simulink library "nonlinearPlant_ul"  (R2018a)
settings: Solver=VariableStepAuto  StartTime=0.0  StopTime=10.0  RelTol=1e-3
values from neighbouring files (symbols this model uses):
  headingTimeConstant_s = 1    [nonlinearPlant_init.m]
  initialHeading_deg = 0    [nonlinearPlant_init.m]
  initialSpeed_mPs = 0    [nonlinearPlant_init.m]
  speedTimeConstant_s = 1    [nonlinearPlant_init.m]
settings Model: Creator=mcobb  LastModifiedBy=mcobb

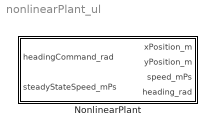
== system nonlinearPlant_ul ==
  NonlinearPlant : Subsystem

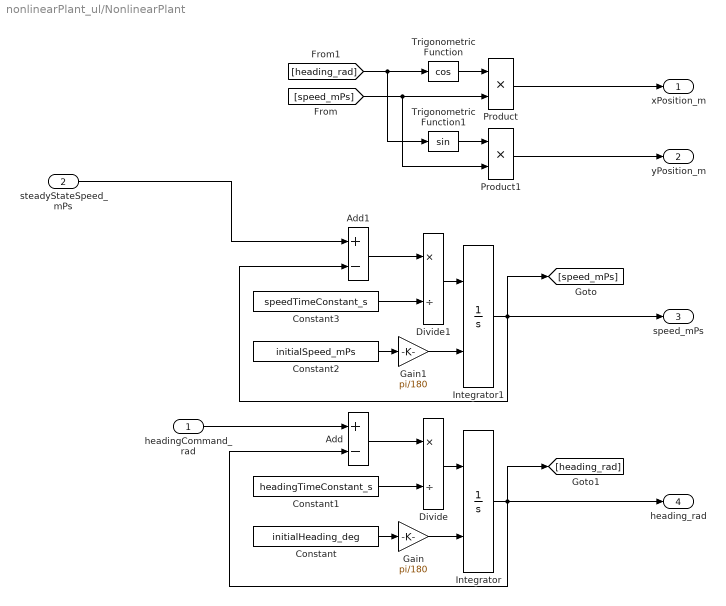
== system nonlinearPlant_ul/NonlinearPlant ==
  headingCommand_rad : Inport
  steadyStateSpeed_mPs : Inport  Port=2
  Add : Sum  Inputs=+-
  Add1 : Sum  Inputs=+-
  Constant : Constant  Value=initialHeading_deg
  Constant1 : Constant  Value=headingTimeConstant_s
  Constant2 : Constant  Value=initialSpeed_mPs
  Constant3 : Constant  Value=speedTimeConstant_s
  Divide : Product  Inputs=*/
  Divide1 : Product  Inputs=*/
  Gain : Gain  Gain=pi/180
  Gain1 : Gain  Gain=pi/180
  Integrator : Integrator  InitialConditionSource=external
  Integrator1 : Integrator  InitialConditionSource=external
  Product : Product
  Product1 : Product
  Trigonometric Function : Trigonometry  Operator=cos
  Trigonometric Function1 : Trigonometry
  xPosition_m : Outport
  yPosition_m : Outport  Port=2
  speed_mPs : Outport  Port=3
  heading_rad : Outport  Port=4
  wires:
  Trigonometric Function/1 -> Product/1
  [heading_rad] -> Trigonometric Function/1, Trigonometric Function1/1
  Product/1 -> xPosition_m/1
  Product1/1 -> yPosition_m/1
  [speed_mPs] -> Product1/2, Product/2
  Trigonometric Function1/1 -> Product1/1
  Constant/1 -> Gain/1
  Gain/1 -> Integrator/2
  Constant1/1 -> Divide/2
  Add/1 -> Divide/1
  Divide/1 -> Integrator/1
  Integrator/1 -> [heading_rad], heading_rad/1, Add/2
  headingCommand_rad/1 -> Add/1
  steadyStateSpeed_mPs/1 -> Add1/1
  Integrator1/1 -> [speed_mPs], speed_mPs/1, Add1/2
  Divide1/1 -> Integrator1/1
  Add1/1 -> Divide1/1
  Constant3/1 -> Divide1/2
  Gain1/1 -> Integrator1/2
  Constant2/1 -> Gain1/1
